simulink model "IM_panel_3"  (R2019b)
settings: Solver=ode45  StartTime=0.0  StopTime=2  RelTol=1e-6  AbsTol=1e-8
values from neighbouring files (symbols this model uses):
  B = 0.08    [IM_Mainprog.m]
  Hc = 1/Kpc    (= 0.063526309481)    [IM_Mainprog.m]
  i_r_alpha_0 = 0    [IM_Mainprog.m]
  i_r_beta_0 = 0    [IM_Mainprog.m]
  i_s_alpha_0 = 0    [IM_Mainprog.m]
  i_s_beta_0 = 0    [IM_Mainprog.m]
  J = 0.01275    [IM_Mainprog.m]
  Kic = alpha_c*(Ra + R_r + R_s)    (= 15741.509434)    [IM_Mainprog.m]
  Kpc = alpha_c * L_sigma    (= 15.741509434)    [IM_Mainprog.m]
  L_M = L_m^2 / L_r    (= 0.127358490566)    [IM_Mainprog.m]
  L_m = 135e-3    (= 0.135)    [IM_Mainprog.m]
  L_r = Lr_lambda + L_m    (= 0.1431)    [IM_Mainprog.m]
  L_s = Ls_lambda + L_m    (= 0.1431)    [IM_Mainprog.m]
  L_sigma = L_s - ((L_m)*(L_m)/L_r)    (= 0.015741509434)    [IM_Mainprog.m]
  np = 2    [IM_Mainprog.m]
  omega_r_0 = 0    [IM_Mainprog.m]
  Psi_ref = 0.8867    [IM_Mainprog.m]
  Psi_ref_time = 1e-3    (= 0.001)    [IM_Mainprog.m]
  R_r = 1.24    [IM_Mainprog.m]
  R_R = (L_m/L_r)^2 * R_r    (= 1.10359558562)    [IM_Mainprog.m]
  R_s = 1.33    [IM_Mainprog.m]
  Ra = L_sigma* alpha_c - R_s - R_r    (= 13.171509434)    [IM_Mainprog.m]
  Teref1 = 12    [IM_Mainprog.m]
  Teref1_time = 1    [IM_Mainprog.m]
  Teref2 = 8    [IM_Mainprog.m]
  Teref2_time = 2    [IM_Mainprog.m]
  Teref3 = 8    [IM_Mainprog.m]
  Teref3_time = 2.1    [IM_Mainprog.m]
  theta_r_0 = 0    [IM_Mainprog.m]
  Tstep = 0    [IM_Mainprog.m]
  Tstep_time = 0    [IM_Mainprog.m]
  usd0 = sqrt(2)*230    [IM_Mainprog.m]
  usq0 = 0    [IM_Mainprog.m]
  VconvLim = 440 * sqrt(2/3)    [IM_Mainprog.m]
  ws = 2*pi*50    (= 314.159265359)    [IM_Mainprog.m]
undefined symbols (not defined in the file or in its folder): j
settings Model: ExtModeTrigMode=oneshot  ExtModeArmWhenConnect=off  ExtModeAutoUpdateStatusClock=off  Creator=e6zebra  LastModifiedBy=smitd
settings SolverCC: AutoScaleAbsTol=off
settings DataIOCC: SaveFormat=Array  SignalLoggingSaveFormat=ModelDataLogs  ReturnWorkspaceOutputs=off
settings OptimizationCC: BlockReduction=off  BooleanDataType=off  ExpressionDepthLimit=2147483647  InitFltsAndDblsToZero=on  LifeSpan=inf
settings DebuggingCC: SaveWithParameterizedLinksMsg=none  UnderspecifiedInitializationDetection=Classic  MergeDetectMultiDrivingBlocksExec=none  SignalResolutionControl=TryResolveAllWithWarning  MultiTaskDSMMsg=warning  MultiTaskCondExecSysMsg=none  FcnCallInpInsideContextMsg=warning  StateNameClashWarn=warning  SFUnexpectedBacktrackingDiag=warning  SFNoUnconditionalDefaultTransitionDiag=warning  SFExecutionAtInitializationDiag=none  ArithmeticOperatorsInVariantConditions=warning
settings HardwareCC: ProdBitPerPointer=32  ProdBitPerSizeT=32  ProdBitPerPtrDiffT=32  ProdLargestAtomicFloat=None  ProdIntDivRoundTo=Undefined  ProdEndianess=Unspecified  ProdWordSize=32  ProdHWDeviceType=32-bit Generic  TargetUnknown=on
settings ModelReferenceCC: PropagateSignalLabelsOutOfModel=off
settings SFSimCC: SimUseLocalCustomCode=off  CustomCodeUndefinedFunction=UseInterfaceOnly
settings RTWCC: TemplateMakefile=grt.tmf  RTWUseLocalCustomCode=off
settings CodeAppCC: StateflowObjectComments=on
settings GRTTargetCC: TargetFcnLib=ansi_tfl_tmw.mat  TargetLangStandard=C89/C90 (ANSI)  GeneratePreprocessorConditionals=Disable all  CombineOutputUpdateFcns=off  GRTInterface=on
settings ConfigComp: CovMetricSettings=dw  CovHtmlReporting=on  CovSaveCumulativeToWorkspaceVar=on  CovSaveSingleToWorkspaceVar=on  CovExternalEMLEnable=off  CovSFcnEnable=off

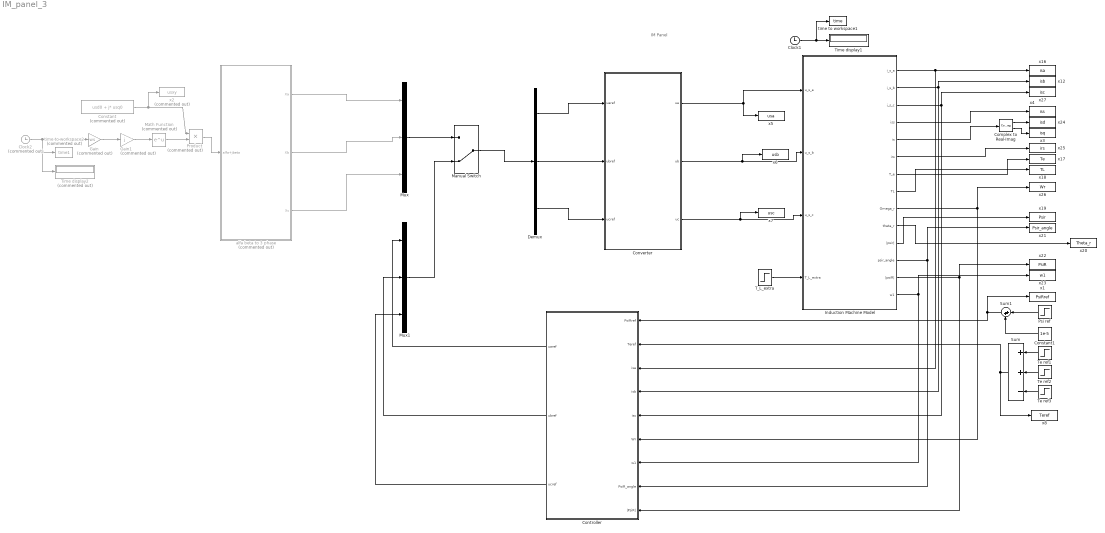
== system IM_panel_3 ==
  note: IM Panel
  Clock1 : Clock
  Clock2 : Clock  Commented=on
  Complex to Real-Imag : ComplexToRealImag
  Constant : Constant  Commented=on  Value=usd0 + j* usq0
  Constant1 : Constant  Value=1e-5
  Controller : Subsystem
  Converter : Subsystem
  Demux : Demux  Outputs=3
  Gain : Gain  Commented=on  Gain=ws
  Gain1 : Gain  Commented=on  Gain=j
  Induction Machine Model : Subsystem
  Manual Switch : ManualSwitch  CurrentSetting=0
  Math Function : Math  Commented=on  SignedPower=off  SaturateOnIntegerOverflow=on
  Mux : Mux  Inputs=3
  Mux1 : Mux  Inputs=3
  Product : Product  Commented=on
  Psi ref : Step  Time=Psi_ref_time  After=Psi_ref  SampleTime=0
  Sum : Sum  Inputs=++-
  Sum1 : Sum  Inputs=|++
  T_L_extra : Step  Time=Tstep_time  After=Tstep  SampleTime=0
  Te ref1 : Step  Time=Teref1_time  After=Teref1  SampleTime=0
  Te ref2 : Step  Time=Teref2_time  After=Teref2  SampleTime=0
  Te ref3 : Step  Time=Teref3_time  After=Teref3  SampleTime=0
  Time display1 : Display
  Time display2 : Display  Commented=on
  alfa beta to 3 phase : Subsystem  Commented=on
  time to workspace1 : ToWorkspace  VariableName=time  SampleTime=-1
  time to workspace2 : ToWorkspace  Commented=on  VariableName=time1  SampleTime=-1
  x1 : ToWorkspace  VariableName=PsiRref  SampleTime=-1
  x12 : ToWorkspace  VariableName=isb  SampleTime=-1
  x16 : ToWorkspace  VariableName=isa  SampleTime=-1
  x17 : ToWorkspace  VariableName=Te  SampleTime=-1
  x18 : ToWorkspace  VariableName=TL  SampleTime=-1
  x19 : ToWorkspace  VariableName=Psir  SampleTime=-1
  x2 : ToWorkspace  Commented=on  VariableName=usxy  SampleTime=-1
  x20 : ToWorkspace  VariableName=Theta_r  SampleTime=-1
  x21 : ToWorkspace  VariableName=Psir_angle  SampleTime=-1
  x22 : ToWorkspace  VariableName=PsiR  SampleTime=-1
  x23 : ToWorkspace  VariableName=w1  SampleTime=-1
  x24 : ToWorkspace  VariableName=isd  SampleTime=-1
  x25 : ToWorkspace  VariableName=irs  SampleTime=-1
  x26 : ToWorkspace  VariableName=Wr  SampleTime=-1
  x27 : ToWorkspace  VariableName=isc  SampleTime=-1
  x3 : ToWorkspace  VariableName=isq  SampleTime=-1
  x4 : ToWorkspace  VariableName=iss  SampleTime=-1
  x5 : ToWorkspace  VariableName=usa  SampleTime=-1
  x6 : ToWorkspace  VariableName=usb  SampleTime=-1
  x7 : ToWorkspace  VariableName=usc  SampleTime=-1
  x8 : ToWorkspace  VariableName=Teref  SampleTime=-1
  wires:
  Te ref1/1 -> Sum/1
  Te ref2/1 -> Sum/2
  Te ref3/1 -> Sum/3
  Sum/1 -> Controller/2(Teref), x8/1
  Clock1/1 -> time to workspace1/1, Time display1/1
  Converter/2(ub) -> x6/1, Induction Machine Model/2(u_s_b)
  Induction Machine Model/14(w1) -> Controller/7(w1), x23/1
  Induction Machine Model/11(|psir|) -> x19/1
  Induction Machine Model/12(psir_angle) -> Controller/8(PsiR_angle), x21/1
  Induction Machine Model/13(|psiR|) -> Controller/9(|PsiR|), x22/1
  Induction Machine Model/10(theta_r) -> x20/1
  Induction Machine Model/4(iss) -> x4/1
  Induction Machine Model/9(Omega_r) -> Controller/6(Wr), x26/1
  Converter/3(uc) -> x7/1, Induction Machine Model/3(u_s_c)
  Induction Machine Model/7(T_e) -> x17/1
  Induction Machine Model/6(irs) -> x25/1
  Converter/1(ua) -> Induction Machine Model/1(u_s_a), x5/1
  Induction Machine Model/8(TL) -> x18/1
  T_L_extra/1 -> Induction Machine Model/4(T_L_extra)
  Induction Machine Model/1(i_s_a) -> Controller/3(isa), x16/1
  Induction Machine Model/2(i_s_b) -> Controller/4(isb), x12/1
  Induction Machine Model/3(i_s_c) -> Controller/5(isc), x27/1
  Gain/1 -> Gain1/1
  Clock2/1 -> Time display2/1, time to workspace2/1, Gain/1
  Product/1 -> alfa beta to 3 phase/1(alfa+jbeta)
  Gain1/1 -> Math Function/1
  Math Function/1 -> Product/2
  Constant/1 -> Product/1, x2/1
  Complex to Real-Imag/1 -> x24/1
  Complex to Real-Imag/2 -> x3/1
  Induction Machine Model/5(is) -> Complex to Real-Imag/1
  alfa beta to 3 phase/1(Xa) -> Mux/1
  alfa beta to 3 phase/2(Xb) -> Mux/2
  alfa beta to 3 phase/3(Xc) -> Mux/3
  Mux1/1 -> Manual Switch/2
  Mux/1 -> Manual Switch/1
  Manual Switch/1 -> Demux/1
  Demux/1 -> Converter/1(uaref)
  Demux/2 -> Converter/2(ubref)
  Demux/3 -> Converter/3(ucref)
  Psi ref/1 -> Sum1/1
  Constant1/1 -> Sum1/2
  Sum1/1 -> Controller/1(PsiRref), x1/1
  Controller/1(uaref) -> Mux1/1
  Controller/2(ubref) -> Mux1/2
  Controller/3(ucref) -> Mux1/3

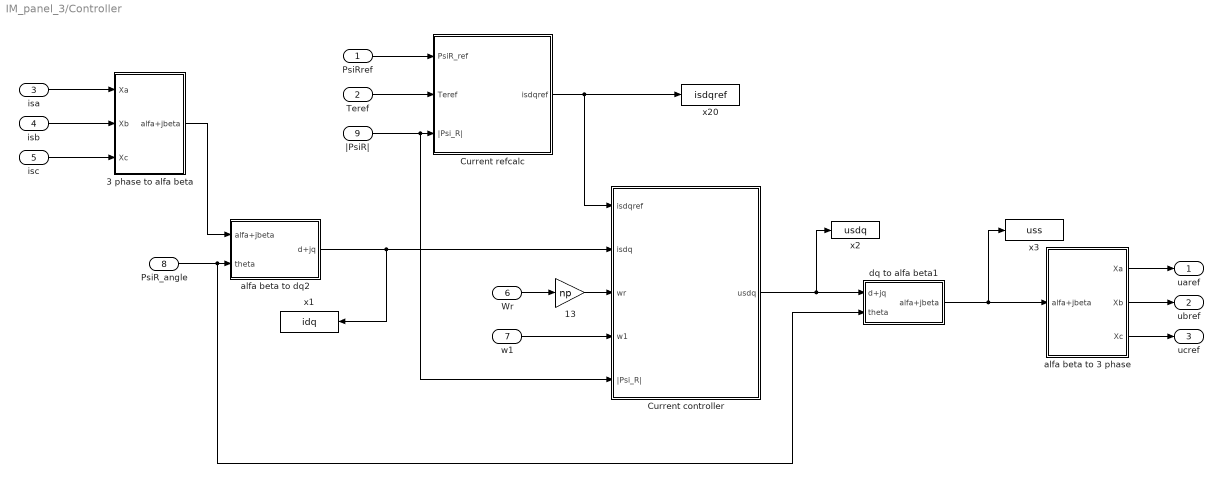
== system IM_panel_3/Controller ==
  PsiRref : Inport
  Teref : Inport  Port=2
  isa : Inport  Port=3
  isb : Inport  Port=4
  isc : Inport  Port=5
  Wr : Inport  Port=6
  w1 : Inport  Port=7
  PsiR_angle : Inport  Port=8
  |PsiR| : Inport  Port=9
  " 13" : Gain  Gain=np
  3 phase to alfa beta : Subsystem
  Current controller : Subsystem
  Current refcalc : Subsystem
  alfa beta to 3 phase : Subsystem
  alfa beta to dq2 : Subsystem
  dq to alfa beta1 : Subsystem
  x1 : ToWorkspace  VariableName=idq  SampleTime=-1
  x2 : ToWorkspace  VariableName=usdq  SampleTime=-1
  x20 : ToWorkspace  VariableName=isdqref  SampleTime=-1
  x3 : ToWorkspace  VariableName=uss  SampleTime=-1
  uaref : Outport  VectorParamsAs1DForOutWhenUnconnected=off
  ubref : Outport  Port=2  VectorParamsAs1DForOutWhenUnconnected=off
  ucref : Outport  Port=3  VectorParamsAs1DForOutWhenUnconnected=off
  wires:
  isa/1 -> 3 phase to alfa beta/1(Xa)
  isb/1 -> 3 phase to alfa beta/2(Xb)
  isc/1 -> 3 phase to alfa beta/3(Xc)
  3 phase to alfa beta/1(alfa+jbeta) -> alfa beta to dq2/1(alfa+jbeta)
  PsiR_angle/1 -> dq to alfa beta1/2(theta), alfa beta to dq2/2(theta)
  PsiRref/1 -> Current refcalc/1(PsiR_ref)
  Teref/1 -> Current refcalc/2(Teref)
  |PsiR|/1 -> Current controller/5(|Psi_R|), Current refcalc/3(|Psi_R|)
  Current refcalc/1(isdqref) -> Current controller/1(isdqref), x20/1
  alfa beta to dq2/1(d+jq) -> x1/1, Current controller/2(isdq)
  dq to alfa beta1/1(alfa+jbeta) -> x3/1, alfa beta to 3 phase/1(alfa+jbeta)
  alfa beta to 3 phase/1(Xa) -> uaref/1
  alfa beta to 3 phase/2(Xb) -> ubref/1
  alfa beta to 3 phase/3(Xc) -> ucref/1
  w1/1 -> Current controller/4(w1)
  Current controller/1(usdq) -> x2/1, dq to alfa beta1/1(d+jq)
  Wr/1 -> " 13"/1
  " 13"/1 -> Current controller/3(wr)

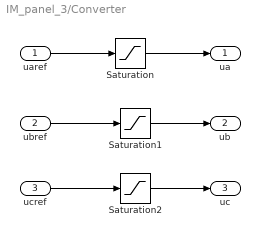
== system IM_panel_3/Converter ==
  uaref : Inport
  ubref : Inport  Port=2
  ucref : Inport  Port=3
  Saturation : Saturate  UpperLimit=VconvLim  LowerLimit=-VconvLim
  Saturation1 : Saturate  UpperLimit=VconvLim  LowerLimit=-VconvLim
  Saturation2 : Saturate  UpperLimit=VconvLim  LowerLimit=-VconvLim
  ua : Outport  VectorParamsAs1DForOutWhenUnconnected=off
  ub : Outport  Port=2  VectorParamsAs1DForOutWhenUnconnected=off
  uc : Outport  Port=3  VectorParamsAs1DForOutWhenUnconnected=off
  wires:
  Saturation2/1 -> uc/1
  Saturation1/1 -> ub/1
  Saturation/1 -> ua/1
  uaref/1 -> Saturation/1
  ubref/1 -> Saturation1/1
  ucref/1 -> Saturation2/1

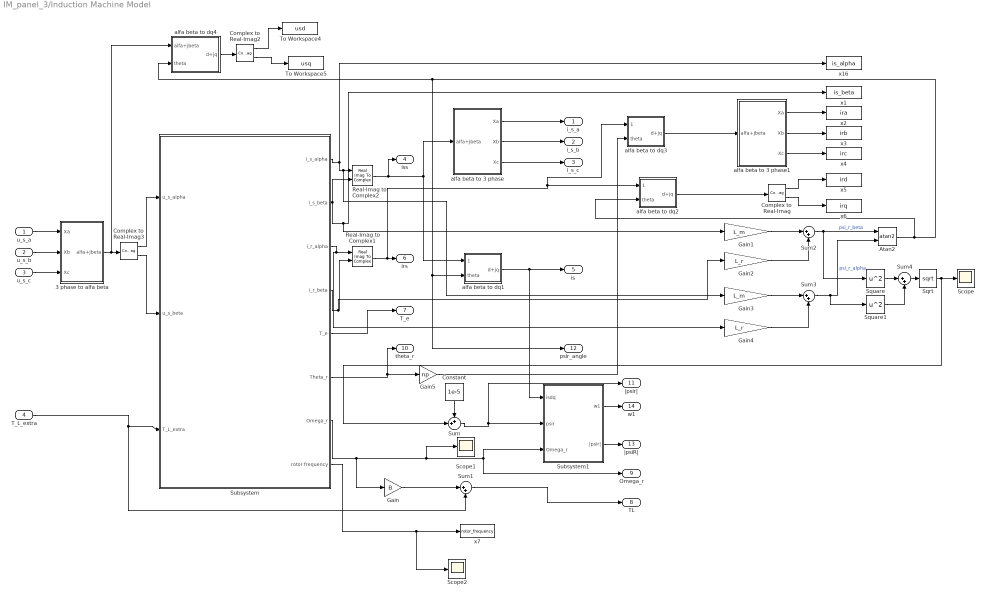
== system IM_panel_3/Induction Machine Model ==
  u_s_a : Inport
  u_s_b : Inport  Port=2
  u_s_c : Inport  Port=3
  T_L_extra : Inport  Port=4
  3 phase to alfa beta : Subsystem
  Atan2 : Trigonometry  Operator=atan2
  Complex to Real-Imag : ComplexToRealImag
  Complex to Real-Imag2 : ComplexToRealImag
  Complex to Real-Imag3 : ComplexToRealImag
  Constant : Constant  Value=1e-5
  Gain : Gain  Gain=B
  Gain1 : Gain  Gain=L_m
  Gain2 : Gain  Gain=L_r
  Gain3 : Gain  Gain=L_m
  Gain4 : Gain  Gain=L_r
  Gain5 : Gain  Gain=np
  Real-Imag to Complex1 : RealImagToComplex
  Real-Imag to Complex2 : RealImagToComplex
  Scope : Scope
  Scope1 : Scope
  Scope2 : Scope
  Sqrt : Sqrt  SaturateOnIntegerOverflow=on
  Square : Math  Operator=square  SignedPower=off  SaturateOnIntegerOverflow=on
  Square1 : Math  Operator=square  SignedPower=off  SaturateOnIntegerOverflow=on
  Subsystem : Subsystem
  Subsystem1 : Subsystem
  Sum : Sum  Inputs=++|
  Sum{1..4} (4 alike) : Sum  Inputs=|++
  To Workspace4 : ToWorkspace  VariableName=usd  SampleTime=-1
  To Workspace5 : ToWorkspace  VariableName=usq  SampleTime=-1
  alfa beta to 3 phase : Subsystem
  alfa beta to 3 phase1 : Subsystem
  alfa beta to dq1 : Subsystem
  alfa beta to dq2 : Subsystem
  alfa beta to dq3 : Subsystem
  alfa beta to dq4 : Subsystem
  x1 : ToWorkspace  VariableName=is_beta  SampleTime=-1
  x16 : ToWorkspace  VariableName=is_alpha  SampleTime=-1
  x2 : ToWorkspace  VariableName=ira  SampleTime=-1
  x3 : ToWorkspace  VariableName=irb  SampleTime=-1
  x4 : ToWorkspace  VariableName=irc  SampleTime=-1
  x5 : ToWorkspace  VariableName=ird  SampleTime=-1
  x6 : ToWorkspace  VariableName=irq  SampleTime=-1
  x7 : ToWorkspace  VariableName=rotor_frequency  SampleTime=-1
  i_s_a : Outport  VectorParamsAs1DForOutWhenUnconnected=off
  i_s_b : Outport  Port=2  VectorParamsAs1DForOutWhenUnconnected=off
  i_s_c : Outport  Port=3  VectorParamsAs1DForOutWhenUnconnected=off
  iss : Outport  Port=4  VectorParamsAs1DForOutWhenUnconnected=off
  is : Outport  Port=5  VectorParamsAs1DForOutWhenUnconnected=off
  irs : Outport  Port=6  VectorParamsAs1DForOutWhenUnconnected=off
  T_e : Outport  Port=7  VectorParamsAs1DForOutWhenUnconnected=off
  TL : Outport  Port=8  VectorParamsAs1DForOutWhenUnconnected=off
  Omega_r : Outport  Port=9  VectorParamsAs1DForOutWhenUnconnected=off
  theta_r : Outport  Port=10  VectorParamsAs1DForOutWhenUnconnected=off
  |psir| : Outport  Port=11  VectorParamsAs1DForOutWhenUnconnected=off
  psir_angle : Outport  Port=12  VectorParamsAs1DForOutWhenUnconnected=off
  |psiR| : Outport  Port=13  VectorParamsAs1DForOutWhenUnconnected=off
  w1 : Outport  Port=14  VectorParamsAs1DForOutWhenUnconnected=off
  wires:
  u_s_a/1 -> 3 phase to alfa beta/1(Xa)
  u_s_b/1 -> 3 phase to alfa beta/2(Xb)
  u_s_c/1 -> 3 phase to alfa beta/3(Xc)
  3 phase to alfa beta/1(alfa+jbeta) -> alfa beta to dq4/1(alfa+jbeta), Complex to Real-Imag3/1
  Real-Imag to Complex2/1 -> alfa beta to 3 phase/1(alfa+jbeta), alfa beta to dq1/1(alfa+jbeta), iss/1
  alfa beta to 3 phase/1(Xa) -> i_s_a/1
  alfa beta to 3 phase/2(Xb) -> i_s_b/1
  alfa beta to 3 phase/3(Xc) -> i_s_c/1
  Complex to Real-Imag3/1 -> Subsystem/1(u_s_alpha)
  Complex to Real-Imag3/2 -> Subsystem/2(u_s_beta)
  T_L_extra/1 -> Sum1/2, Subsystem/3(T_L_extra)
  Subsystem/1(i_s_alpha) -> x16/1, Gain3/1, Real-Imag to Complex2/1
  Subsystem/3(i_r_alpha) -> Gain4/1, Real-Imag to Complex1/1
  Subsystem/4(i_r_beta) -> Gain2/1, Real-Imag to Complex1/2
  Subsystem/5(T_e) -> T_e/1
  Subsystem/6(Theta_r) -> theta_r/1, Gain5/1
  Constant/1 -> Sum/1
  alfa beta to dq1/1(d+jq) -> Subsystem1/1(isdq), is/1
  Sqrt/1 -> Scope/1, Sum/2
  Sum1/1 -> TL/1
  Gain/1 -> Sum1/1
  Subsystem1/1(w1) -> w1/1
  Subsystem1/2(|psir|) -> |psiR|/1
  Subsystem/7(Omega_r) -> Gain/1, Scope1/1, Subsystem1/3(Omega_r), Omega_r/1
  Subsystem/2(i_s_beta) -> Gain1/1, x1/1, Real-Imag to Complex2/2
  alfa beta to 3 phase1/1(Xa) -> x2/1
  alfa beta to 3 phase1/2(Xb) -> x3/1
  alfa beta to 3 phase1/3(Xc) -> x4/1
  Sum/1 -> |psir|/1, Subsystem1/2(psir)
  Sum4/1 -> Sqrt/1
  Square/1 -> Sum4/1
  Gain3/1 -> Sum3/1
  Square1/1 -> Sum4/2
  Sum3/1 -> Square1/1, Atan2/2  "psi_r_alpha"
  Gain4/1 -> Sum3/2
  Sum2/1 -> Square/1, Atan2/1  "psi_r_beta"
  Gain2/1 -> Sum2/2
  Gain1/1 -> Sum2/1
  Real-Imag to Complex1/1 -> alfa beta to dq3/1(alfa+jbeta), alfa beta to dq2/1(alfa+jbeta), irs/1
  alfa beta to dq2/1(d+jq) -> Complex to Real-Imag/1
  Complex to Real-Imag/1 -> x5/1
  Complex to Real-Imag/2 -> x6/1
  alfa beta to dq3/1(d+jq) -> alfa beta to 3 phase1/1(alfa+jbeta)
  Gain5/1 -> alfa beta to dq3/2(theta)
  Complex to Real-Imag2/1 -> To Workspace4/1
  alfa beta to dq4/1(d+jq) -> Complex to Real-Imag2/1
  Complex to Real-Imag2/2 -> To Workspace5/1
  Atan2/1 -> alfa beta to dq2/2(theta), alfa beta to dq4/2(theta), psir_angle/1, alfa beta to dq1/2(theta)
  Subsystem/8(rotor frequency) -> Scope2/1, x7/1

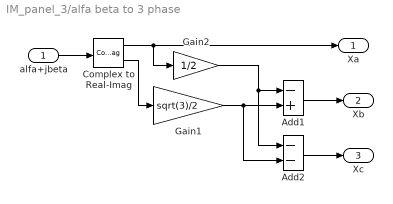
== system IM_panel_3/alfa beta to 3 phase ==
  alfa+jbeta : Inport
  Add1 : Sum  Inputs=-+
  Add2 : Sum  Inputs=--
  Complex to Real-Imag : ComplexToRealImag
  Gain1 : Gain  Gain=sqrt(3)/2
  Gain2 : Gain  Gain=1/2
  Xa : Outport  VectorParamsAs1DForOutWhenUnconnected=off
  Xb : Outport  Port=2  VectorParamsAs1DForOutWhenUnconnected=off
  Xc : Outport  Port=3  VectorParamsAs1DForOutWhenUnconnected=off
  wires:
  alfa+jbeta/1 -> Complex to Real-Imag/1
  Complex to Real-Imag/1 -> Xa/1, Gain2/1
  Add2/1 -> Xc/1
  Add1/1 -> Xb/1
  Complex to Real-Imag/2 -> Gain1/1
  Gain1/1 -> Add1/2, Add2/2
  Gain2/1 -> Add1/1, Add2/1

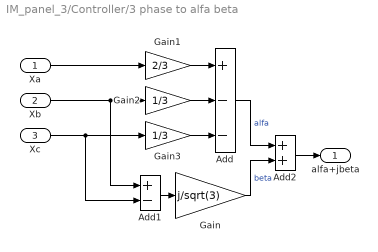
== system IM_panel_3/Controller/3 phase to alfa beta ==
  Xa : Inport
  Xb : Inport  Port=2
  Xc : Inport  Port=3
  Add : Sum  Inputs=+--
  Add1 : Sum  Inputs=+-
  Add2 : Sum
  Gain : Gain  Gain=j/sqrt(3)
  Gain1 : Gain  Gain=2/3
  Gain2 : Gain  Gain=1/3
  Gain3 : Gain  Gain=1/3
  alfa+jbeta : Outport  VectorParamsAs1DForOutWhenUnconnected=off
  wires:
  Add1/1 -> Gain/1
  Add2/1 -> alfa+jbeta/1
  Gain/1 -> Add2/2  "beta"
  Add/1 -> Add2/1  "alfa"
  Gain3/1 -> Add/3
  Gain2/1 -> Add/2
  Gain1/1 -> Add/1
  Xa/1 -> Gain1/1
  Xb/1 -> Gain2/1, Add1/1
  Xc/1 -> Gain3/1, Add1/2

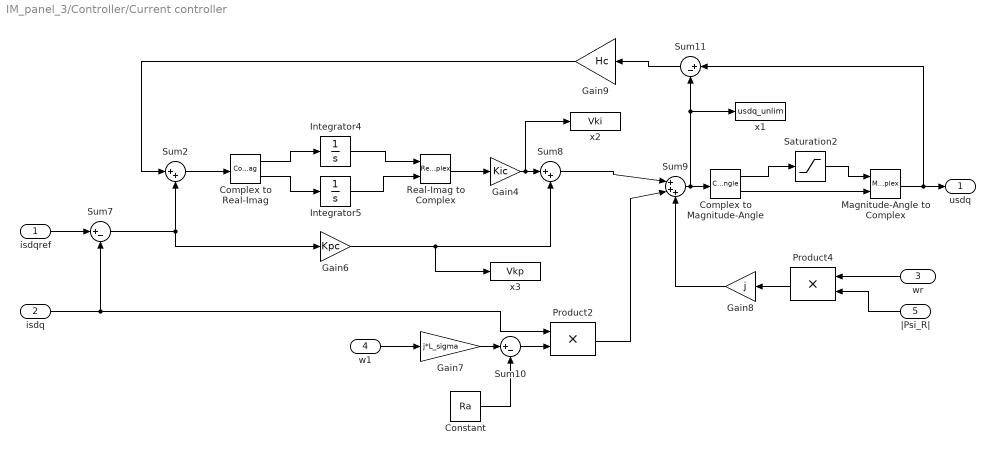
== system IM_panel_3/Controller/Current controller ==
  isdqref : Inport
  isdq : Inport  Port=2
  wr : Inport  Port=3
  w1 : Inport  Port=4
  |Psi_R| : Inport  Port=5
  Complex to Magnitude-Angle : ComplexToMagnitudeAngle
  Complex to Real-Imag : ComplexToRealImag
  Constant : Constant  Value=Ra
  Gain4 : Gain  Gain=Kic
  Gain6 : Gain  Gain=Kpc
  Gain7 : Gain  Gain=j*L_sigma
  Gain8 : Gain  Gain=j
  Gain9 : Gain  Gain=Hc
  Integrator4 : Integrator
  Integrator5 : Integrator
  Magnitude-Angle to Complex : MagnitudeAngleToComplex
  Product2 : Product  SaturateOnIntegerOverflow=on  OutDataTypeStr=Inherit: Same as first input
  Product4 : Product  SaturateOnIntegerOverflow=on  OutDataTypeStr=Inherit: Same as first input
  Real-Imag to Complex : RealImagToComplex
  Saturation2 : Saturate  UpperLimit=VconvLim  LowerLimit=-VconvLim
  Sum10 : Sum  Inputs=|+-
  Sum11 : Sum  Inputs=|+-
  Sum2 : Sum  Inputs=|++
  Sum7 : Sum  Inputs=|+-
  Sum8 : Sum  Inputs=|++
  Sum9 : Sum  Inputs=|+++
  x1 : ToWorkspace  VariableName=usdq_unlim  SampleTime=-1
  x2 : ToWorkspace  VariableName=Vki  SampleTime=-1
  x3 : ToWorkspace  VariableName=Vkp  SampleTime=-1
  usdq : Outport  VectorParamsAs1DForOutWhenUnconnected=off
  wires:
  isdqref/1 -> Sum7/1
  isdq/1 -> Product2/1, Sum7/2
  Sum7/1 -> Gain6/1, Sum2/2
  Sum2/1 -> Complex to Real-Imag/1
  Complex to Real-Imag/1 -> Integrator4/1
  Complex to Real-Imag/2 -> Integrator5/1
  Integrator4/1 -> Real-Imag to Complex/1
  Integrator5/1 -> Real-Imag to Complex/2
  Real-Imag to Complex/1 -> Gain4/1
  Gain4/1 -> x2/1, Sum8/1
  Gain6/1 -> x3/1, Sum8/2
  Sum8/1 -> Sum9/1
  w1/1 -> Gain7/1
  Gain7/1 -> Sum10/1
  Constant/1 -> Sum10/2
  Sum10/1 -> Product2/2
  Product2/1 -> Sum9/2
  Product4/1 -> Gain8/1
  wr/1 -> Product4/1
  |Psi_R|/1 -> Product4/2
  Gain8/1 -> Sum9/3
  Sum9/1 -> x1/1, Sum11/2, Complex to Magnitude-Angle/1
  Complex to Magnitude-Angle/1 -> Saturation2/1
  Saturation2/1 -> Magnitude-Angle to Complex/1
  Complex to Magnitude-Angle/2 -> Magnitude-Angle to Complex/2
  Magnitude-Angle to Complex/1 -> Sum11/1, usdq/1
  Sum11/1 -> Gain9/1
  Gain9/1 -> Sum2/1

== system IM_panel_3/Controller/Current refcalc ==
  PsiR_ref : Inport
  Teref : Inport  Port=2
  |Psi_R| : Inport  Port=3
  " 15" : Gain  Gain=1/L_M
  " 16" : Gain  Gain=2/(3*np)
  Divide1 : Product  Inputs=*/
  Real-Imag to Complex : RealImagToComplex
  isdqref : Outport  VectorParamsAs1DForOutWhenUnconnected=off
  wires:
  PsiR_ref/1 -> " 15"/1
  " 15"/1 -> Real-Imag to Complex/1
  Teref/1 -> Divide1/1
  |Psi_R|/1 -> Divide1/2
  Divide1/1 -> " 16"/1  "w2"
  " 16"/1 -> Real-Imag to Complex/2
  Real-Imag to Complex/1 -> isdqref/1

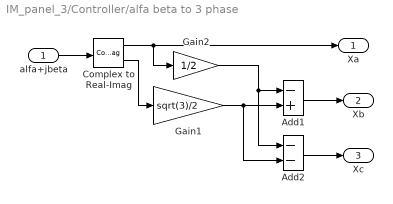
== system IM_panel_3/Controller/alfa beta to 3 phase ==
  alfa+jbeta : Inport
  Add1 : Sum  Inputs=-+
  Add2 : Sum  Inputs=--
  Complex to Real-Imag : ComplexToRealImag
  Gain1 : Gain  Gain=sqrt(3)/2
  Gain2 : Gain  Gain=1/2
  Xa : Outport  VectorParamsAs1DForOutWhenUnconnected=off
  Xb : Outport  Port=2  VectorParamsAs1DForOutWhenUnconnected=off
  Xc : Outport  Port=3  VectorParamsAs1DForOutWhenUnconnected=off
  wires:
  alfa+jbeta/1 -> Complex to Real-Imag/1
  Complex to Real-Imag/1 -> Xa/1, Gain2/1
  Add2/1 -> Xc/1
  Add1/1 -> Xb/1
  Complex to Real-Imag/2 -> Gain1/1
  Gain1/1 -> Add1/2, Add2/2
  Gain2/1 -> Add1/1, Add2/1

== system IM_panel_3/Controller/alfa beta to dq2 ==
  alfa+jbeta : Inport
  theta : Inport  Port=2
  Gain : Gain  Gain=-j  SaturateOnIntegerOverflow=on  OutDataTypeStr=Inherit: Same as input  ParamDataTypeStr=Inherit: Same as input
  Math Function : Math  SaturateOnIntegerOverflow=on
  Product : Product  SaturateOnIntegerOverflow=on  OutDataTypeStr=Inherit: Same as first input
  d+jq : Outport  VectorParamsAs1DForOutWhenUnconnected=off
  wires:
  theta/1 -> Gain/1
  Gain/1 -> Math Function/1
  Math Function/1 -> Product/2
  alfa+jbeta/1 -> Product/1
  Product/1 -> d+jq/1

== system IM_panel_3/Controller/dq to alfa beta1 ==
  d+jq : Inport
  theta : Inport  Port=2
  Gain : Gain  Gain=j  SaturateOnIntegerOverflow=on  OutDataTypeStr=Inherit: Same as input  ParamDataTypeStr=Inherit: Same as input
  Math Function : Math  SaturateOnIntegerOverflow=on
  Product : Product  SaturateOnIntegerOverflow=on  OutDataTypeStr=Inherit: Same as first input
  alfa+jbeta : Outport  VectorParamsAs1DForOutWhenUnconnected=off
  wires:
  theta/1 -> Gain/1
  Gain/1 -> Math Function/1
  Math Function/1 -> Product/2
  d+jq/1 -> Product/1
  Product/1 -> alfa+jbeta/1

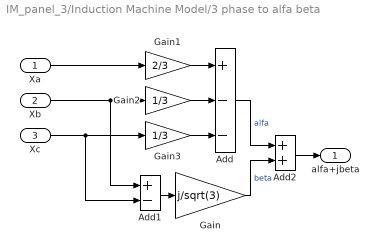
== system IM_panel_3/Induction Machine Model/3 phase to alfa beta ==
  Xa : Inport
  Xb : Inport  Port=2
  Xc : Inport  Port=3
  Add : Sum  Inputs=+--
  Add1 : Sum  Inputs=+-
  Add2 : Sum
  Gain : Gain  Gain=j/sqrt(3)
  Gain1 : Gain  Gain=2/3
  Gain2 : Gain  Gain=1/3
  Gain3 : Gain  Gain=1/3
  alfa+jbeta : Outport  VectorParamsAs1DForOutWhenUnconnected=off
  wires:
  Add1/1 -> Gain/1
  Add2/1 -> alfa+jbeta/1
  Gain/1 -> Add2/2  "beta"
  Add/1 -> Add2/1  "alfa"
  Gain3/1 -> Add/3
  Gain2/1 -> Add/2
  Gain1/1 -> Add/1
  Xa/1 -> Gain1/1
  Xb/1 -> Gain2/1, Add1/1
  Xc/1 -> Gain3/1, Add1/2

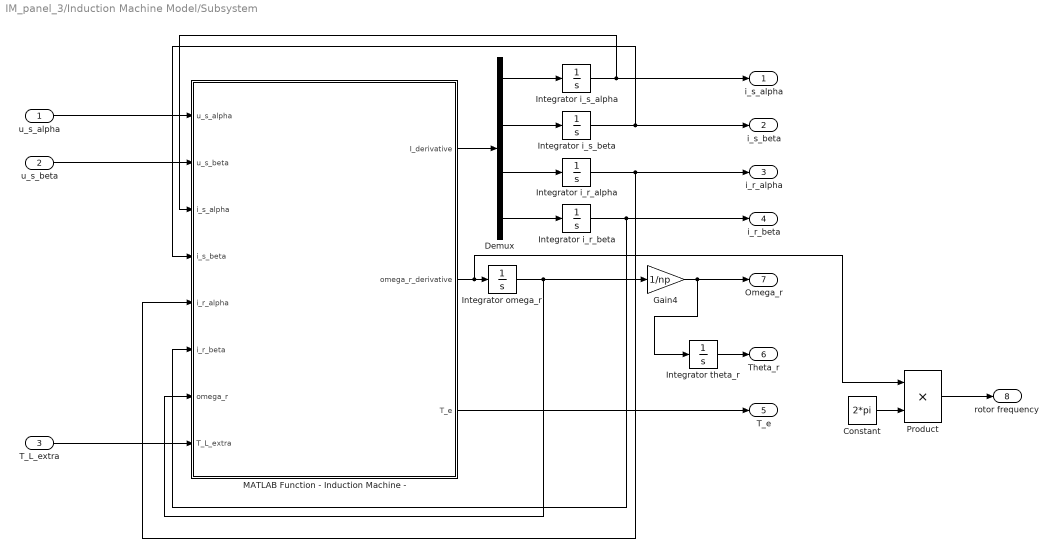
== system IM_panel_3/Induction Machine Model/Subsystem ==
  u_s_alpha : Inport
  u_s_beta : Inport  Port=2
  T_L_extra : Inport  Port=3
  Constant : Constant  Value=2*pi
  Demux : Demux
  Gain4 : Gain  Gain=1/np
  Integrator i_r_alpha : Integrator  InitialCondition=i_r_alpha_0
  Integrator i_r_beta : Integrator  InitialCondition=i_r_beta_0
  Integrator i_s_alpha : Integrator  InitialCondition=i_s_alpha_0
  Integrator i_s_beta : Integrator  InitialCondition=i_s_beta_0
  Integrator omega_r : Integrator  InitialCondition=omega_r_0
  Integrator theta_r : Integrator  InitialCondition=theta_r_0  WrapState=on
  MATLAB Function - Induction Machine - : MATLAB Function  TreatAsAtomicUnit=on
  Product : Product
  i_s_alpha : Outport
  i_s_beta : Outport  Port=2
  i_r_alpha : Outport  Port=3
  i_r_beta : Outport  Port=4
  T_e : Outport  Port=5  VectorParamsAs1DForOutWhenUnconnected=off
  Theta_r : Outport  Port=6  VectorParamsAs1DForOutWhenUnconnected=off
  Omega_r : Outport  Port=7
  rotor frequency : Outport  Port=8  VectorParamsAs1DForOutWhenUnconnected=off
  wires:
  MATLAB Function - Induction Machine -/1(I_derivative) -> Demux/1
  Integrator i_r_alpha/1 -> i_r_alpha/1, MATLAB Function - Induction Machine -/5(i_r_alpha)
  Demux/4 -> Integrator i_r_beta/1
  Integrator i_s_beta/1 -> MATLAB Function - Induction Machine -/4(i_s_beta), i_s_beta/1
  u_s_beta/1 -> MATLAB Function - Induction Machine -/2(u_s_beta)
  Demux/2 -> Integrator i_s_beta/1
  Demux/1 -> Integrator i_s_alpha/1
  Integrator i_s_alpha/1 -> MATLAB Function - Induction Machine -/3(i_s_alpha), i_s_alpha/1
  MATLAB Function - Induction Machine -/3(T_e) -> T_e/1
  T_L_extra/1 -> MATLAB Function - Induction Machine -/8(T_L_extra)
  Demux/3 -> Integrator i_r_alpha/1
  u_s_alpha/1 -> MATLAB Function - Induction Machine -/1(u_s_alpha)
  Integrator theta_r/1 -> Theta_r/1
  Integrator i_r_beta/1 -> i_r_beta/1, MATLAB Function - Induction Machine -/6(i_r_beta)
  MATLAB Function - Induction Machine -/2(omega_r_derivative) -> Product/1, Integrator omega_r/1
  Integrator omega_r/1 -> Gain4/1, MATLAB Function - Induction Machine -/7(omega_r)
  Gain4/1 -> Integrator theta_r/1, Omega_r/1
  Constant/1 -> Product/2
  Product/1 -> rotor frequency/1

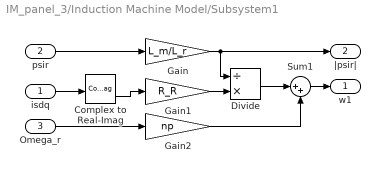
== system IM_panel_3/Induction Machine Model/Subsystem1 ==
  isdq : Inport
  psir : Inport  Port=2
  Omega_r : Inport  Port=3
  Complex to Real-Imag : ComplexToRealImag
  Divide : Product  Inputs=/*
  Gain : Gain  Gain=L_m/L_r
  Gain1 : Gain  Gain=R_R
  Gain2 : Gain  Gain=np
  Sum1 : Sum  Inputs=|++
  w1 : Outport
  |psir| : Outport  Port=2
  wires:
  Gain/1 -> |psir|/1, Divide/1
  Gain1/1 -> Divide/2
  Sum1/1 -> w1/1
  Divide/1 -> Sum1/1
  Omega_r/1 -> Gain2/1
  Gain2/1 -> Sum1/2
  isdq/1 -> Complex to Real-Imag/1
  Complex to Real-Imag/2 -> Gain1/1
  psir/1 -> Gain/1

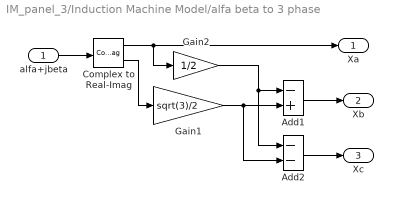
== system IM_panel_3/Induction Machine Model/alfa beta to 3 phase ==
  alfa+jbeta : Inport
  Add1 : Sum  Inputs=-+
  Add2 : Sum  Inputs=--
  Complex to Real-Imag : ComplexToRealImag
  Gain1 : Gain  Gain=sqrt(3)/2
  Gain2 : Gain  Gain=1/2
  Xa : Outport  VectorParamsAs1DForOutWhenUnconnected=off
  Xb : Outport  Port=2  VectorParamsAs1DForOutWhenUnconnected=off
  Xc : Outport  Port=3  VectorParamsAs1DForOutWhenUnconnected=off
  wires:
  alfa+jbeta/1 -> Complex to Real-Imag/1
  Complex to Real-Imag/1 -> Xa/1, Gain2/1
  Add2/1 -> Xc/1
  Add1/1 -> Xb/1
  Complex to Real-Imag/2 -> Gain1/1
  Gain1/1 -> Add1/2, Add2/2
  Gain2/1 -> Add1/1, Add2/1

== system IM_panel_3/Induction Machine Model/alfa beta to 3 phase1 ==
  alfa+jbeta : Inport
  Add1 : Sum  Inputs=-+
  Add2 : Sum  Inputs=--
  Complex to Real-Imag : ComplexToRealImag
  Gain1 : Gain  Gain=sqrt(3)/2
  Gain2 : Gain  Gain=1/2
  Xa : Outport  VectorParamsAs1DForOutWhenUnconnected=off
  Xb : Outport  Port=2  VectorParamsAs1DForOutWhenUnconnected=off
  Xc : Outport  Port=3  VectorParamsAs1DForOutWhenUnconnected=off
  wires:
  Gain2/1 -> Add2/1, Add1/1
  Gain1/1 -> Add2/2, Add1/2
  Complex to Real-Imag/2 -> Gain1/1
  Add1/1 -> Xb/1
  Add2/1 -> Xc/1
  Complex to Real-Imag/1 -> Gain2/1, Xa/1
  alfa+jbeta/1 -> Complex to Real-Imag/1

== system IM_panel_3/Induction Machine Model/alfa beta to dq1 ==
  alfa+jbeta : Inport
  theta : Inport  Port=2
  Gain : Gain  Gain=-j  SaturateOnIntegerOverflow=on  OutDataTypeStr=Inherit: Same as input  ParamDataTypeStr=Inherit: Same as input
  Math Function : Math  SaturateOnIntegerOverflow=on
  Product : Product  SaturateOnIntegerOverflow=on  OutDataTypeStr=Inherit: Same as first input
  d+jq : Outport  VectorParamsAs1DForOutWhenUnconnected=off
  wires:
  theta/1 -> Gain/1
  Gain/1 -> Math Function/1
  Math Function/1 -> Product/2
  alfa+jbeta/1 -> Product/1
  Product/1 -> d+jq/1

== system IM_panel_3/Induction Machine Model/alfa beta to dq2 ==
  alfa+jbeta : Inport
  theta : Inport  Port=2
  Gain : Gain  Gain=-j  SaturateOnIntegerOverflow=on  OutDataTypeStr=Inherit: Same as input  ParamDataTypeStr=Inherit: Same as input
  Math Function : Math  SaturateOnIntegerOverflow=on
  Product : Product  SaturateOnIntegerOverflow=on  OutDataTypeStr=Inherit: Same as first input
  d+jq : Outport  VectorParamsAs1DForOutWhenUnconnected=off
  wires:
  Product/1 -> d+jq/1
  alfa+jbeta/1 -> Product/1
  Math Function/1 -> Product/2
  Gain/1 -> Math Function/1
  theta/1 -> Gain/1

== system IM_panel_3/Induction Machine Model/alfa beta to dq3 ==
  alfa+jbeta : Inport
  theta : Inport  Port=2
  Gain : Gain  Gain=-j  SaturateOnIntegerOverflow=on  OutDataTypeStr=Inherit: Same as input  ParamDataTypeStr=Inherit: Same as input
  Math Function : Math  SaturateOnIntegerOverflow=on
  Product : Product  SaturateOnIntegerOverflow=on  OutDataTypeStr=Inherit: Same as first input
  d+jq : Outport  VectorParamsAs1DForOutWhenUnconnected=off
  wires:
  Product/1 -> d+jq/1
  alfa+jbeta/1 -> Product/1
  Math Function/1 -> Product/2
  Gain/1 -> Math Function/1
  theta/1 -> Gain/1

== system IM_panel_3/Induction Machine Model/alfa beta to dq4 ==
  alfa+jbeta : Inport
  theta : Inport  Port=2
  Gain : Gain  Gain=-j  SaturateOnIntegerOverflow=on  OutDataTypeStr=Inherit: Same as input  ParamDataTypeStr=Inherit: Same as input
  Math Function : Math  SaturateOnIntegerOverflow=on
  Product : Product  SaturateOnIntegerOverflow=on  OutDataTypeStr=Inherit: Same as first input
  d+jq : Outport  VectorParamsAs1DForOutWhenUnconnected=off
  wires:
  theta/1 -> Gain/1
  Gain/1 -> Math Function/1
  Math Function/1 -> Product/2
  alfa+jbeta/1 -> Product/1
  Product/1 -> d+jq/1

== matlab function IM_panel_3/Induction Machine Model/Subsystem/MATLAB Function - Induction Machine - ==
  data: I_derivative output; omega_r_derivative output; u_s_alpha input; T_e output; u_s_beta input; i_s_alpha input; i_s_beta input; i_r_alpha input; i_r_beta input; omega_r input; T_L_extra input; np parameter; R_s parameter; R_r parameter; L_s parameter; L_r parameter; L_m parameter; B parameter; J parameter
function [ I_derivative , omega_r_derivative , T_e ] = ...
    induction_machine_function( u_s_alpha , u_s_beta , i_s_alpha , i_s_beta, i_r_alpha , i_r_beta , omega_r , T_L_extra , np , R_s , R_r , L_s , L_r , L_m , B , J )
% Description
% Standard syntax of funtion in MATLAB:
% funtion [ function_outputs ] = ( function_inputs )
% please use the same variable names as given in the inputs and outputs of
% the function

%% Electrical Derivatives
R_matrix = [R_s             0               0               0; 
            0               R_s             0               0;
            0               omega_r*L_m     R_r             omega_r*L_r;
            -omega_r*L_m    0               -omega_r*L_r    R_r];    
          
L_matrix = [L_s 0   L_m 0;
            0   L_s 0   L_m;
            L_m 0   L_r 0; 
            0   L_m 0   L_r];           
          
I_array = [ i_s_alpha ; i_s_beta ; i_r_alpha ; i_r_beta];
U_array = [ u_s_alpha ; u_s_beta ;         0 ;        0];

% I_derivative =-L_matrix\R_matrix*I_array + L_matrix\U_array;
I_derivative = (-inv(L_matrix)*R_matrix*I_array) + (inv(L_matrix)*U_array);

%% Mechanical Derivatives

% Electromagnetic Torque
T_e = 3/2 * np * L_m * ((i_r_alpha* i_s_beta)- (i_r_beta*i_s_alpha));

% Load Torque
T_L = (B * omega_r/np) + T_L_extra;

% Electromagnetic Torque
omega_r_derivative = np  * ((T_e - T_L)/J);

end
